simulink model "DataGenerator2DOF"  (R2018b)
settings: Solver=FixedStepAuto  StartTime=0.0  StopTime=20  FixedStep=0.008  RelTol=1e-3
settings Model: Creator=root  LastModifiedBy=root

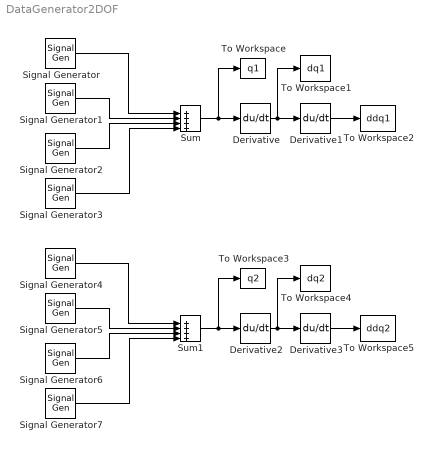
== system DataGenerator2DOF ==
  Derivative{,1..3} (4 alike) : Derivative
  Signal Generator : SignalGenerator  Frequency=0.5  Units=rad/sec
  Signal Generator1 : SignalGenerator  Units=rad/sec
  Signal Generator2 : SignalGenerator  Frequency=1.5  Units=rad/sec
  Signal Generator3 : SignalGenerator  Frequency=2  Units=rad/sec
  Signal Generator4 : SignalGenerator  Amplitude=-1  Frequency=0.5  Units=rad/sec
  Signal Generator5 : SignalGenerator  Amplitude=-1  Units=rad/sec
  Signal Generator6 : SignalGenerator  Amplitude=-1  Frequency=1.5  Units=rad/sec
  Signal Generator7 : SignalGenerator  Amplitude=-1  Frequency=2  Units=rad/sec
  Sum : Sum  Inputs=|++++
  Sum1 : Sum  Inputs=|++++
  To Workspace : ToWorkspace  VariableName=q1  SampleTime=0.008
      settings: Save2DSignal=2-D array (concatenate along first dimension)
  To Workspace1 : ToWorkspace  VariableName=dq1  SampleTime=0.008
      settings: Save2DSignal=2-D array (concatenate along first dimension)
  To Workspace2 : ToWorkspace  VariableName=ddq1  SampleTime=0.008
      settings: Save2DSignal=2-D array (concatenate along first dimension)
  To Workspace3 : ToWorkspace  VariableName=q2  SampleTime=0.008
      settings: Save2DSignal=2-D array (concatenate along first dimension)
  To Workspace4 : ToWorkspace  VariableName=dq2  SampleTime=0.008
      settings: Save2DSignal=2-D array (concatenate along first dimension)
  To Workspace5 : ToWorkspace  VariableName=ddq2  SampleTime=0.008
      settings: Save2DSignal=2-D array (concatenate along first dimension)
  wires:
  Signal Generator/1 -> Sum/1
  Signal Generator1/1 -> Sum/2
  Signal Generator2/1 -> Sum/3
  Signal Generator3/1 -> Sum/4
  Derivative/1 -> Derivative1/1, To Workspace1/1
  Derivative1/1 -> To Workspace2/1
  Signal Generator4/1 -> Sum1/1
  Sum1/1 -> To Workspace3/1, Derivative2/1
  Signal Generator7/1 -> Sum1/4
  Signal Generator5/1 -> Sum1/2
  Signal Generator6/1 -> Sum1/3
  Derivative2/1 -> Derivative3/1, To Workspace4/1
  Derivative3/1 -> To Workspace5/1
  Sum/1 -> To Workspace/1, Derivative/1
